simulink model "maximum_power"  (R2023b)
settings: Solver=VariableStepAuto  StartTime=0.0  StopTime=stepp.sim_time*2  RelTol=1e-3
values from neighbouring files (symbols this model uses):
  Bat =     [Samsung_30Q_18650_pack.mat]
undefined symbols (not defined in the file or in its folder): boost, Ci, Ion, KR, Lithium, m0_ccm, mppt_my2, pv_data, pv_eq, Ramp, Ru, sim_op, Ti
libraries: spsSeriesRLCBranchLib x6, spsCurrentMeasurementLib x3, spsVoltageMeasurementLib x3, spsBatteryLib x1, spsDiodeLib x1, spsControlledCurrentSourceLib x1, spsIdealSwitchLib x1, simulink_extras x1, spsBistableLib x1, slpidlib x1, sps_lib x1
settings Model: Creator=teo  LastModifiedBy=teo
settings SolverCC: ZeroCrossAlgorithm=Adaptive
settings DebuggingCC: IgnoredZcDiagnostic=none

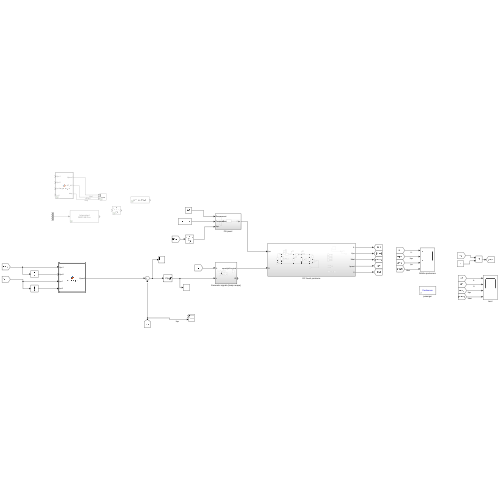
[thumbnail: Simulink's stored preview of the top-level diagram]
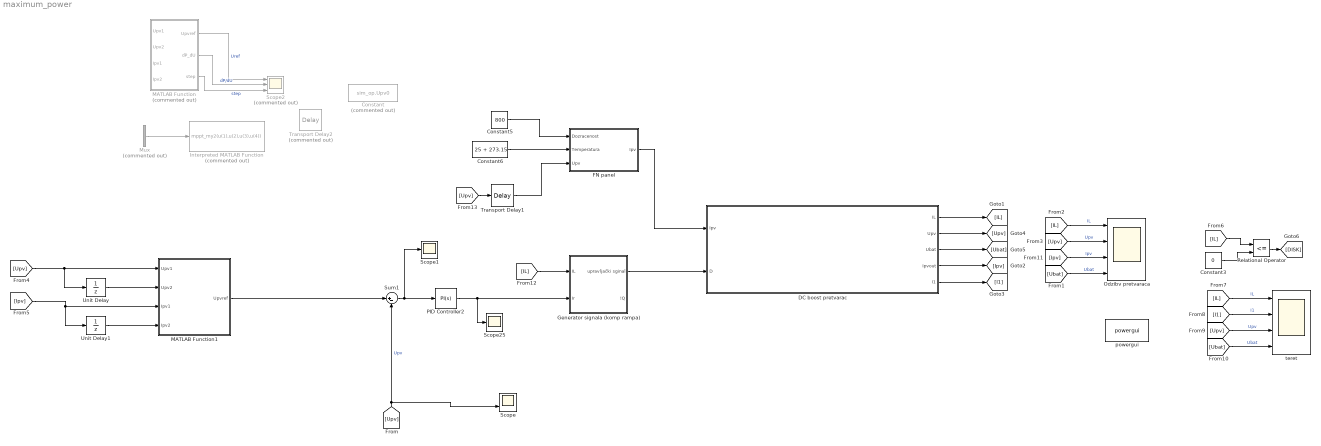
== system maximum_power ==
  Constant : Constant  Commented=on  Value=sim_op.Upv0
  Constant3 : Constant  Value=0
  Constant5 : Constant  Value=800
  Constant6 : Constant  Value=25 + 273.15
  DC boost pretvarac : Subsystem
  FN panel : Subsystem
  Generator signala (komp rampa) : Subsystem
  Interpreted MATLAB Function : MATLABFcn  Commented=on  MATLABFcn=mppt_my2(u(1),u(2),u(3),u(4))
  MATLAB Function : MATLAB Function  Commented=on  TreatAsAtomicUnit=on
  MATLAB Function1 : MATLAB Function  TreatAsAtomicUnit=on
  Mux : Mux  Commented=on
  Odzibv pretvaraca : Scope  NumInputPorts=4
  PID Controller2 : slpidlib/PID Controller  Controller=PI  Form=Parallel  TimeDomain=Continuous-time  UseExternalTs=off  SampleTime=-1  IntegratorMethod=Forward Euler  FilterMethod=Forward Euler  ControllerParametersSource=internal  P=KR  I=KR/Ti  UseKiTs=off  D=0  N=100  UseFilter=on  TunerSelectOption=Transfer Function Based (PID Tuner App)  InitialConditionSource=internal  InitialConditionForIntegrator=0  InitialConditionForFilter=0  DifferentiatorICPrevScaledInput=0  ExternalReset=none  TrackingMode=off  Kt=1  LimitOutput=on  SatLimitsSource=internal  UpperSaturationLimit=1.9  LowerSaturationLimit=-1.9  LinearizeAsGain=off  AntiWindupMode=clamping  Kb=1  LimitIntegrator=off  UpperIntegratorSaturationLimit=inf  LowerIntegratorSaturationLimit=-inf  POutMin=[]  POutMax=[]  IOutMin=[]  IOutMax=[]  DOutMin=[]  DOutMax=[]  NOutMin=[]  NOutMax=[]  SumOutMin=[]  SumOutMax=[]  SaturationOutMin=[]  SaturationOutMax=[]  PParamMin=[]  PParamMax=[]  IParamMin=[]  IParamMax=[]  DParamMin=[]  DParamMax=[]  NParamMin=[]  NParamMax=[]  KbParamMin=[]  KbParamMax=[]  KtParamMin=[]  KtParamMax=[]  KbOutMin=[]  KbOutMax=[]  KtOutMin=[]  KtOutMax=[]  IntegratorOutMin=[]  IntegratorOutMax=[]  FilterOutMin=[]  FilterOutMax=[]  SumI1OutMin=[]  SumI1OutMax=[]  SumI2OutMin=[]  SumI2OutMax=[]  SumI3OutMin=[]  SumI3OutMax=[]  SumI4OutMin=[]  SumI4OutMax=[]  SumDOutMin=[]  SumDOutMax=[]  DifferentiatorOutMin=[]  DifferentiatorOutMax=[]  FilterDiffOutCoefMin=[]  FilterDiffOutCoefMax=[]  ReciprocalOutMin=[]  ReciprocalOutMax=[]  SumDenOutMin=[]  SumDenOutMax=[]  SumNumOutMin=[]  SumNumOutMax=[]  DivideOutMin=[]  DivideOutMax=[]  UdiffTsProdOutMin=[]  UdiffTsProdOutMax=[]  NTsProdOutMin=[]  NTsProdOutMax=[]  UintegralTsProdOutMin=[]  UintegralTsProdOutMax=[]  UngainTsProdOutMin=[]  UngainTsProdOutMax=[]  ClampingZeroOutDataTypeStr=Inherit: Inherit via back propagation  ClampingZeroOutMin=[]  ClampingZeroOutMax=[]  FilterDenConstantOutDataTypeStr=Inherit: Inherit via back propagation  FilterDenConstantOutMin=[]  FilterDenConstantOutMax=[]  PCopyOutDataTypeStr=Inherit: Inherit via back propagation  PCopyOutMin=[]  PCopyOutMax=[]  NCopyOutDataTypeStr=Inherit: Inherit via back propagation  NCopyOutMin=[]  NCopyOutMax=[]  IntegratorContinuousStateAttributes=''  IntegratorStateMustResolveToSignalObject=off  IntegratorRTWStateStorageClass=Auto  FilterContinuousStateAttributes=''  FilterStateMustResolveToSignalObject=off  FilterRTWStateStorageClass=Auto  ParallelPVariant=InternalParameters  IdealPVariant=Disabled  IVariant=InternalParameters  DVariant=Disabled  IntegratorVariant=Continuous  SatVariant=Enabled  AWVariant=ContClampingParallel  PCopyVariant=Disabled  TRVariant=Disabled  FdbkBlocksVariant=Forward  IdealPFdbkVariant=Disabled  SatFdbkVariant=Disabled  DerivativeFilterVariant=Disabled  NVariant=Disabled  NCopyVariant=Disabled_SignalSpec  FilterICVariant=Disabled  IntegratorICVariant=InternalICs  ExternalResetVariant=Disabled  TRSumVariant=Passthrough  SumFdbkVariant=Disabled  SumVariant=Sum_PI  TsampFilterVariant=InternalTs  TsampNgainVariant=Passthrough  TsampIntegralVariant=Disabled_SignalSpec  ExternalSaturationOutDataTypeStr=Inherit: Same as second input
  Relational Operator : RelationalOperator  Operator=<=  OutDataTypeStr=boolean  RndMeth=Simplest  InputSameDT=off
  Scope : Scope  NumInputPorts=2
  Scope1 : Scope
  Scope2 : Scope  Commented=on  NumInputPorts=3
  Scope25 : Scope
  Sum1 : Sum  Inputs=|+-
  Transport Delay1 : TransportDelay  DelayTime=0.0001  BufferSize=4024
  Transport Delay2 : TransportDelay  Commented=on  DelayTime=0.01  BufferSize=4024
  Unit Delay : UnitDelay  SampleTime=-1  HasFrameUpgradeWarning=on
  Unit Delay1 : UnitDelay  SampleTime=-1  HasFrameUpgradeWarning=on
  powergui : sps_lib/powergui  Priority=1  SimulationMode=Continuous  SampleTime=50e-6  frequency=60  Iterations=50  frequencyindice=0  Pbase=100e6  ErrMax=1e-4  UnitsV=kV  UnitsW=MW  buscounter=0  FunctionMessages=off  echomessages=off  EnableUseOfTLC=off  CurrentSourceSwitches=off  DisableSnubberDevices=off  DisableRonSwitches=off  DisableVfSwitches=off  DisplayEquations=off  AutomaticDiscreteSolvers=off  SolverType=Tustin/Backward Euler (TBE)  Interpol=off  ExternalGateDelay=off  methode=off  Ts=100  x0status=blocks  SPID=on  SwTol=0  HookPort=off  NonlinearTolerance=1e-4  nMaxIteration=100  ContinueOnMaxIteration=off  RestoreLinks=warning  ResistiveCurrentMeasurement=off  Frange=[0:2:500]  Ylog=off  Xlog=on  ShowGrid=off  save=off  variable=ZData  structure=0  ZoomFFT=off  StartTime=0.0  cycles=1  DisplayStyle=1  fundamental=60  FreqAxis=off  MaxFrequency=1000  frequencyindicesteady=1  RmsSteady=1  display=off
  teret : Scope  NumInputPorts=4
  wires:
  [IL] -> Generator signala (komp rampa)/1(IL)
  FN panel/1(Ipv) -> DC boost pretvarac/1(Ipv)
  Constant6/1 -> FN panel/2(Temperatura)
  Constant3/1 -> Relational Operator/2
  [Ubat] -> Odzibv pretvaraca/4  "Ubat"
  [IL] -> Odzibv pretvaraca/1  "IL"
  DC boost pretvarac/4(Ipvout) -> [Ipv]
  [Upv] -> teret/3  "Upv"
  Generator signala (komp rampa)/1(upravljački sginal) -> DC boost pretvarac/2(D)
  DC boost pretvarac/5(I1) -> [I1]
  [IL] -> teret/1  "IL"
  DC boost pretvarac/3(Ubat) -> [Ubat]
  Transport Delay1/1 -> FN panel/3(Upv)
  [IL] -> Relational Operator/1
  [I1] -> teret/2  "I1"
  Relational Operator/1 -> [DISK]
  PID Controller2/1 -> Generator signala (komp rampa)/2(Ir), Scope25/1
  [Ubat] -> teret/4  "Ubat"
  DC boost pretvarac/1(IL) -> [IL]
  [Ipv] -> Odzibv pretvaraca/3  "Ipv"
  Sum1/1 -> Scope1/1, PID Controller2/1
  DC boost pretvarac/2(Upv) -> [Upv]
  [Upv] -> Odzibv pretvaraca/2  "Upv"
  [Upv] -> Transport Delay1/1
  [Upv] -> Scope/2, Sum1/2  "Upv"
  [Upv] -> Unit Delay/1, MATLAB Function1/1(Upv1)
  [Ipv] -> Unit Delay1/1, MATLAB Function1/3(Ipv1)
  Constant5/1 -> FN panel/1(Dozracenost)
  Mux/1 -> Interpreted MATLAB Function/1
  MATLAB Function/1(Upvref) -> Scope2/1  "Uref"
  MATLAB Function/2(dP_dU) -> Scope2/2  "dP/dU"
  MATLAB Function/3(step) -> Scope2/3  "step"
  MATLAB Function1/1(Upvref) -> Sum1/1
  Unit Delay1/1 -> MATLAB Function1/4(Ipv2)
  Unit Delay/1 -> MATLAB Function1/2(Upv2)

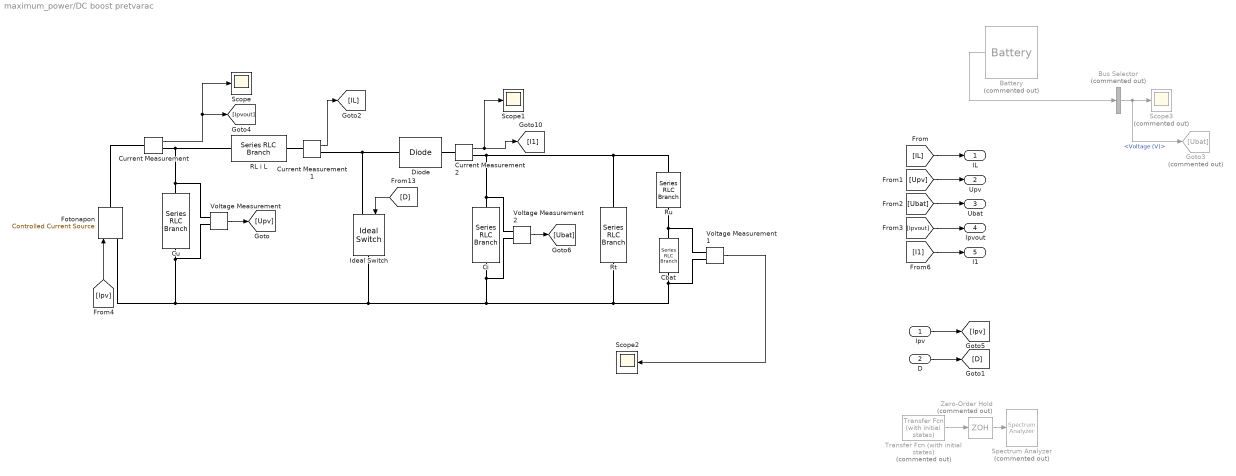
== system maximum_power/DC boost pretvarac ==
  Ipv : Inport
  D : Inport  Port=2
  Battery : spsBatteryLib/Battery  Commented=on  BatType=Lithium-Ion  ShowTempParam=off  ThermalPreset=no  ShowAgeParam=off  NomV=Bat.Ubat_nom  NomQ=Bat.Qbat/1000  SOC=80  Batt_Tr=1e-6  PresetModel=on  MaxQ=3  MinV=8.1  FullV=12.5711  Dis_rate=1.3043  R=0.036  Normal_OP=2.713  expZone="[11.6682     0.147391]"  current=[6.5 13 32.5]  Units=Time  Tci=20  NomT=20  T2=-30  MaxQ2=4.8  FullV2=7.1  Normal_OP2=5.655  expZone2="[6.58           1]"  Rca=0.6  ti=2000  Dp=0  Neq0=0  Tsim=1e6  Ta1=25  Qeol=5.4*0.9  Reol=0.013333*1.2  Char_age=[2.3478, 3]  Dis_age=[2.3478, 10]  N1=1500  N2=10500  N3=1000  N4=1400  Ta2=45  N5=950
  Bus Selector : BusSelector  Commented=on  OutputSignals=Voltage (V)
  Cbat : spsSeriesRLCBranchLib/Series RLC Branch  LConnTagsString=__new0  RConnTagsString=__new0  BranchType=C  Resistance=Ru  Inductance=1e-3  SetiL0=off  InitialCurrent=0  Capacitance=boost.Cbat  Setx0=on  InitialVoltage=sim_op.Ubat0  Measurements=None
  Ci : spsSeriesRLCBranchLib/Series RLC Branch  LConnTagsString=__new0  RConnTagsString=__new0  BranchType=C  Resistance=0.001  Inductance=1e-3  SetiL0=off  InitialCurrent=0  Capacitance=boost.Ci  Setx0=on  InitialVoltage=sim_op.Ubat0  Measurements=None
  Cu : spsSeriesRLCBranchLib/Series RLC Branch  LConnTagsString=__new0  RConnTagsString=__new0  BranchType=C  Resistance=0.001  Inductance=1e-3  SetiL0=off  InitialCurrent=0  Capacitance=boost.Cu  Setx0=on  InitialVoltage=sim_op.Upv0  Measurements=None
  Current Measurement : spsCurrentMeasurementLib/Current Measurement  PhasorSimulation=off  OutputType=Complex  PSBequivalent=0
  Current Measurement1 : spsCurrentMeasurementLib/Current Measurement  PhasorSimulation=off  OutputType=Complex  PSBequivalent=0
  Current Measurement2 : spsCurrentMeasurementLib/Current Measurement  PhasorSimulation=off  OutputType=Complex  PSBequivalent=0
  Diode : spsDiodeLib/Diode  Ron=0  Lon=0  Vf=0  IC=0  UseSnubber=0  Rs=0  Cs=0  Measurements=off
  Fotonapon : spsControlledCurrentSourceLib/Controlled Current Source  Initialize=on  Source_Type=DC  Amplitude=0  Phase=0  Frequency=0  Measurements=None
  Goto3 : Goto  Commented=on  GotoTag=Ubat
  Ideal Switch : spsIdealSwitchLib/Ideal Switch  Ron=0  Lon=0  IC=0  Rs=0  Cs=0  Measurements=off
  RL i L : spsSeriesRLCBranchLib/Series RLC Branch  LConnTagsString=__new0  RConnTagsString=__new0  BranchType=RL  Resistance=boost.RL  Inductance=boost.L  SetiL0=off  InitialCurrent=stepp.ir01  Capacitance=1e-6  Setx0=off  InitialVoltage=0  Measurements=None
  Rt : spsSeriesRLCBranchLib/Series RLC Branch  LConnTagsString=__new0  RConnTagsString=__new0  BranchType=R  Resistance=boost.Rt  Inductance=1e-3  SetiL0=off  InitialCurrent=0  Capacitance=Ci  Setx0=off  InitialVoltage=0  Measurements=None
  Ru : spsSeriesRLCBranchLib/Series RLC Branch  LConnTagsString=__new0  RConnTagsString=__new0  BranchType=R  Resistance=boost.Ru  Inductance=1e-3  SetiL0=off  InitialCurrent=0  Capacitance=Ci  Setx0=on  InitialVoltage=Ubat0_ccm  Measurements=None
  Scope : Scope
  Scope1 : Scope
  Scope2 : Scope
  Scope3 : Scope  Commented=on
  Spectrum Analyzer : SpectrumAnalyzer  Commented=on  WindowPosition=[1.000000,1.000000,1920.000000,1080.000000,]  ScopeFrameLocation=window  Method=Welch  PlotAsTwoSidedSpectrum=off  Span=150000  CenterFrequency=75000  StartFrequency=0  StopFrequency=150000  AveragingMethod=Exponential  ForgettingFactor=1  YLimits=[-162.01370297,70.38685066]  ExpandToolstrip=on  SelectedToolstripTab=spectrumAnalyzerToolstrip.measurementsTab
  Transfer Fcn (with initial states) : simulink_extras/Additional Linear/Transfer Fcn (with initial states)  Commented=on  N=[1]  D=[boost.Tmfc, 1]  X0=.5
  Voltage Measurement : spsVoltageMeasurementLib/Voltage Measurement  PhasorSimulation=off  OutputType=Complex  PSBequivalent=0
  Voltage Measurement1 : spsVoltageMeasurementLib/Voltage Measurement  PhasorSimulation=off  OutputType=Complex  PSBequivalent=0
  Voltage Measurement2 : spsVoltageMeasurementLib/Voltage Measurement  PhasorSimulation=off  OutputType=Complex  PSBequivalent=0
  Zero-Order Hold : ZeroOrderHold  Commented=on  SampleTime=1/(3*boost.f)
  IL : Outport
  Upv : Outport  Port=2
  Ubat : Outport  Port=3
  Ipvout : Outport  Port=4
  I1 : Outport  Port=5
  wires:
  Current Measurement1/1 -> [IL]
  Voltage Measurement/1 -> [Upv]
  [D] -> Ideal Switch/1
  [Ipv] -> Fotonapon/1
  D/1 -> [D]
  Ipv/1 -> [Ipv]
  [IL] -> IL/1
  [Upv] -> Upv/1
  [Ubat] -> Ubat/1
  Current Measurement/1 -> Scope/1, [Ipvout]
  [Ipvout] -> Ipvout/1
  Current Measurement2/1 -> Scope1/1, [I1]
  [I1] -> I1/1
  Voltage Measurement1/1 -> Scope2/1
  Zero-Order Hold/1 -> Spectrum Analyzer/1
  Transfer Fcn (with initial states)/1 -> Zero-Order Hold/1
  Bus Selector/1 -> Goto3/1, Scope3/1  "<Voltage (V)>"
  Battery/1 -> Bus Selector/1
  Voltage Measurement2/1 -> [Ubat]
  connections:
  Current Measurement/RConn1 -- Voltage Measurement/LConn1 -- Cu/LConn1 -- RL i L/LConn1
  RL i L/RConn1 -- Current Measurement1/LConn1
  Diode/LConn1 -- Ideal Switch/LConn1 -- Current Measurement1/RConn1
  Current Measurement2/LConn1 -- Diode/RConn1
  Ci/RConn1 -- Voltage Measurement2/LConn2 -- Voltage Measurement1/LConn2 -- Cbat/RConn1 -- Rt/RConn1 -- Voltage Measurement/LConn2 -- Cu/RConn1 -- Fotonapon/LConn1 -- Ideal Switch/RConn1
  Fotonapon/RConn1 -- Current Measurement/LConn1
  Ci/LConn1 -- Voltage Measurement2/LConn1 -- Ru/LConn1 -- Rt/LConn1 -- Current Measurement2/RConn1
  Ru/RConn1 -- Voltage Measurement1/LConn1 -- Cbat/LConn1

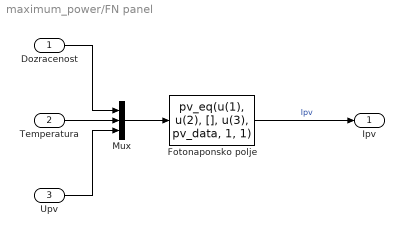
== system maximum_power/FN panel ==
  Dozracenost : Inport
  Temperatura : Inport  Port=2
  Upv : Inport  Port=3
  Fotonaponsko polje : MATLABFcn  MATLABFcn=pv_eq(u(1), u(2), [], u(3), pv_data, 1, 1)  OutputDimensions=1
  Mux : Mux  Inputs=3
  Ipv : Outport
  wires:
  Fotonaponsko polje/1 -> Ipv/1  "Ipv"
  Mux/1 -> Fotonaponsko polje/1
  Dozracenost/1 -> Mux/1
  Temperatura/1 -> Mux/2
  Upv/1 -> Mux/3

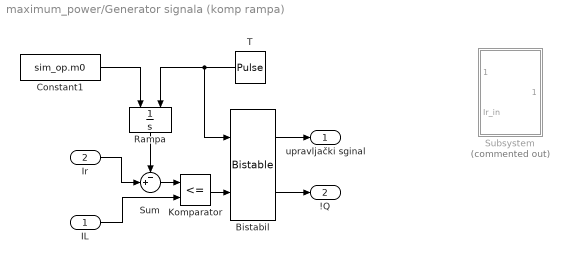
== system maximum_power/Generator signala (komp rampa) ==
  IL : Inport
  Ir : Inport  Port=2
  Bistabil : spsBistableLib/Bistable  Qpriority=Set  ic=0  Ts=0
      settings: LibrarySourceBlock=sps_lib/Control/Bistable
  Constant1 : Constant  Value=sim_op.m0
  Komparator : RelationalOperator  Operator=<=  OutDataTypeStr=boolean  RndMeth=Simplest  InputSameDT=off
  Rampa : Integrator  ExternalReset=rising
  Subsystem : Subsystem  Commented=on
  Sum : Sum  Inputs=-+|
  T : DiscretePulseGenerator  PulseType=Time based  Period=boost.T
  upravljački sginal : Outport
  !Q : Outport  Port=2
  wires:
  Komparator/1 -> Bistabil/2
  Bistabil/2 -> !Q/1
  Bistabil/1 -> upravljački sginal/1
  IL/1 -> Komparator/2
  Sum/1 -> Komparator/1
  Ir/1 -> Sum/2
  Rampa/1 -> Sum/1
  T/1 -> Bistabil/1, Rampa/2
  Constant1/1 -> Rampa/1

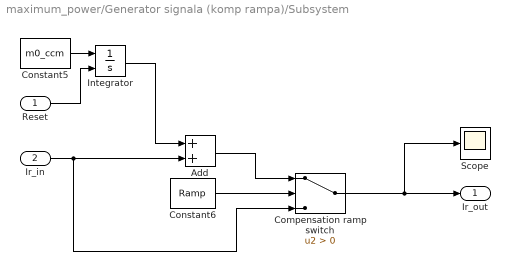
== system maximum_power/Generator signala (komp rampa)/Subsystem ==
  Reset : Inport
  Ir_in : Inport  Port=2
  Add : Sum
  Compensation ramp switch : Switch  Criteria=u2 > Threshold  SaturateOnIntegerOverflow=off  InputSameDT=off
  Constant5 : Constant  Value=m0_ccm
  Constant6 : Constant  Value=Ramp
  Integrator : Integrator  ExternalReset=rising
  Scope : Scope
  Ir_out : Outport
  wires:
  Constant5/1 -> Integrator/1
  Integrator/1 -> Add/1
  Add/1 -> Compensation ramp switch/1
  Reset/1 -> Integrator/2
  Compensation ramp switch/1 -> Scope/1, Ir_out/1
  Constant6/1 -> Compensation ramp switch/2
  Ir_in/1 -> Compensation ramp switch/3, Add/2

== matlab function maximum_power/MATLAB Function1 ==
  data: Upv1 input; Upvref output; Upv2 input; Ipv1 input; Ipv2 input
function Upvref = mppt_my3(Upv1, Upv2, Ipv1, Ipv2)

zero_thresh = 1e-4;
epsilon = 0.01;
step_min = 0.005;
step_max = 0.2;

Upvref = Upv2;

% % Lower bound for safety
% if Upvref < 4
%     Upvref = 4;
%     return;
% elseif Upvref > 6.7
%     Upvref = 6.7;
%     return;
% end
% 
% % Protection: if current is nearly zero → PV not supplying power
% if (Ipv1<zero_thresh)&&(Ipv2<=zero_thresh)
%     Upvref=0.9*Upvref;
%     return;
% end

dUpv = Upv1 - Upv2;
dIpv = Ipv1 - Ipv2;

if (abs(dUpv) < zero_thresh)
    if (abs(dIpv) < zero_thresh)
        return;
    elseif (dIpv > 0)
        Upvref = Upvref + step_min;
        return;
    else 
        Upvref = Upvref - step_min;
        return;
    end
end

Gincr = dIpv/dUpv;
G = Ipv1/Upv1;
dPdU = Gincr + G;

if (abs(dPdU) > epsilon)
    step_var = max(step_min, min(step_max, 5 * abs(dPdU)));
    if (dPdU > 0)
        Upvref = Upvref + step_var;
    else
        Upvref = Upvref - step_var;
    end
end

== matlab function maximum_power/MATLAB Function ==
  data: Upv1 input; Upvref output; Upv2 input; Ipv1 input; Ipv2 input; dP_dU output; step output
function [Upvref, dP_dU, step] = mppt_my2(Upv1, Upv2, Ipv1, Ipv2)

zero_thresh = 1e-3;
epsilon = 0.01;
step_min = 0.005;
step_max = 0.2;

dU = Upv1 - Upv2;
dI = Ipv1 - Ipv2;

Upvref = Upv2;

if Upvref < 4
    Upvref = 4;
end

% Clamp dU to [-2, 2]
dU = max(min(dU, 2), -2);

dP_dU = 0;
step = step_min;
if (abs(dU) < zero_thresh)
    if (abs(dI) < zero_thresh)
        return;
    elseif (dI > 0)
        Upvref = Upvref + step;
    else 
        Upvref = Upvref - step;
    end
    return;
end

if Upv1 < zero_thresh
    Upv1 = zero_thresh;
end

Gincr = dI/dU;
G = Ipv1/Upv1;
dP_dU = Gincr + G;

if (Gincr + G > epsilon)
    % Adaptive step calculation
    scaling = abs(Gincr + G);               % Sensitivity
    scaling = min(max(scaling, 0), 1);      % Clamp to [0, 1]
    step_var = step_min + (step_max - step_min) * scaling;
    step = step_var;
    if (Gincr > -G)
        Upvref = Upvref + step;
    else
        Upvref = Upvref - step;
    end
end

end
